simulink model "simlwrkuka_dynamic_dirdyn"  (R2014a)
settings: Solver=ode1  StartTime=0.0  StopTime=10.0  FixedStep=0.002  RelTol=1e-3
values from neighbouring files (symbols this model uses):
  dqi = [0;0;0;0;0;0;0]    [initial.m]
  qi = [pi/2;0;0;pi/2;0;pi/2;pi/6]    [initial.m]
settings Model: Creator=Admin  LastModifiedBy=faezeh

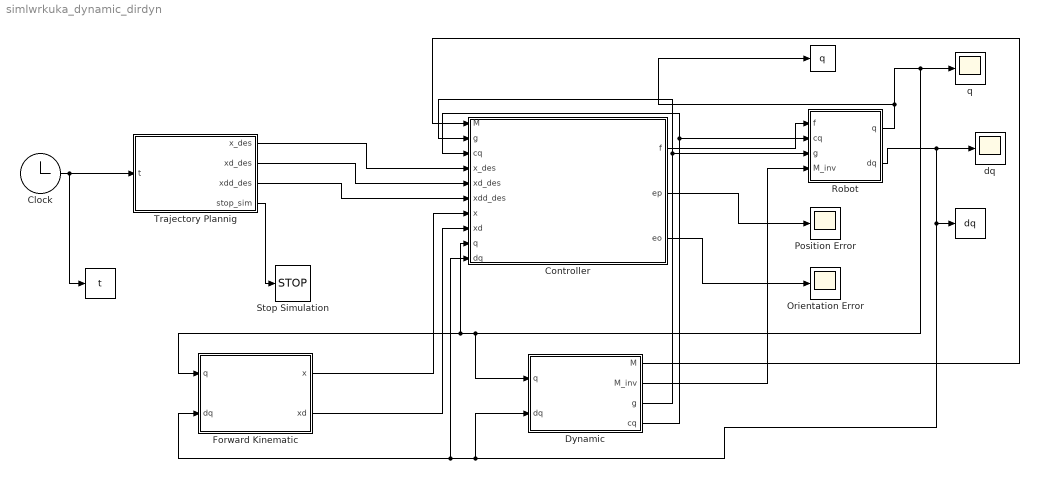
== system simlwrkuka_dynamic_dirdyn ==
  "  " : ToWorkspace  VariableName=q  SampleTime=-1
  "    " : ToWorkspace  VariableName=dq  SampleTime=-1
  "      " : ToWorkspace  VariableName=t  SampleTime=-1
  Clock : Clock
  Controller : MATLAB Function  TreatAsAtomicUnit=on
  Dynamic : MATLAB Function  TreatAsAtomicUnit=on
  Forward Kinematic : MATLAB Function  TreatAsAtomicUnit=on
  Orientation Error : Scope
      settings: SaveName=ScopeData2
  "Position Error " : Scope
  Robot : Subsystem
  Stop Simulation : Stop
  Trajectory Plannig : MATLAB Function  TreatAsAtomicUnit=on
  dq : Scope
      settings: SaveName=ScopeData3
  q : Scope
  wires:
  Clock/1 -> "      "/1, Trajectory Plannig/1(t)
  Trajectory Plannig/4(stop_sim) -> Stop Simulation/1
  Trajectory Plannig/3(xdd_des) -> Controller/6(xdd_des)
  Trajectory Plannig/2(xd_des) -> Controller/5(xd_des)
  Trajectory Plannig/1(x_des) -> Controller/4(x_des)
  Controller/1(f) -> Robot/1(f)
  Controller/2(ep) -> "Position Error "/1
  Controller/3(eo) -> Orientation Error/1
  Robot/1(q) -> Dynamic/1(q), Controller/9(q), Forward Kinematic/1(q), q/1, "  "/1
  Robot/2(dq) -> Dynamic/2(dq), Controller/10(dq), Forward Kinematic/2(dq), "    "/1, dq/1
  Forward Kinematic/1(x) -> Controller/7(x)
  Forward Kinematic/2(xd) -> Controller/8(xd)
  Dynamic/4(cq) -> Robot/2(cq), Controller/3(cq)
  Dynamic/3(g) -> Robot/3(g), Controller/2(g)
  Dynamic/1(M) -> Controller/1(M)
  Dynamic/2(M_inv) -> Robot/4(M_inv)

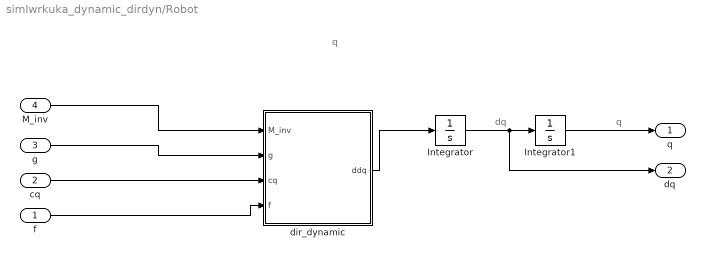
== system simlwrkuka_dynamic_dirdyn/Robot ==
  note: q
  note: q
  note: dq
  f : Inport
  cq : Inport  Port=2
  g : Inport  Port=3
  M_inv : Inport  Port=4
  Integrator : Integrator  InitialCondition=dqi
  Integrator1 : Integrator  InitialCondition=qi
  dir_dynamic : MATLAB Function  TreatAsAtomicUnit=on
  q : Outport
  dq : Outport  Port=2
  wires:
  f/1 -> dir_dynamic/4(f)
  dir_dynamic/1(ddq) -> Integrator/1
  Integrator/1 -> dq/1, Integrator1/1
  Integrator1/1 -> q/1
  g/1 -> dir_dynamic/2(g)
  M_inv/1 -> dir_dynamic/1(M_inv)
  cq/1 -> dir_dynamic/3(cq)

== matlab function simlwrkuka_dynamic_dirdyn/Controller ==
  data: M input; f output; g input; cq input; ep output; eo output; x_des input; xd_des input; xdd_des input; x input; xd input; q input; dq input
function [f,ep,eo] = command(M,g,cq,x_des,xd_des,xdd_des,x,xd,q,dq)
[J,Te]=jacobin(q(1),q(2),q(3),q(4),q(5),q(6),q(7));
Re=Te(1:3,1:3);
kp=15;
kd=10;
kpo=15;
eps=x(5:7);
eta=x(4);
eta_des=x_des(4);
eps_des=x_des(5:7);
S_eps=[0 -eps(3) eps(2); eps(3) 0 -eps(1);-eps(2) eps(1) 0];
eps_de=(eta*eps_des-eta_des*eps-S_eps*eps_des);
xd_com_o=xd_des(4:6)+kpo*Re*eps_de;
xd_com_p=xd_des(1:3)+kp*(x_des(1:3)-x(1:3));
Xd_com=[xd_com_p;xd_com_o];
f=M*pinv(J)*(xdd_des+kd*(xd_des-xd)+Xd_com-xd_des)+cq+g;
ep=x_des(1:3)-x(1:3);
eo=x_des(4:6)-x(4:6);

== matlab function simlwrkuka_dynamic_dirdyn/Trajectory Plannig ==
  data: t input; x_des output; xd_des output; xdd_des output; stop_sim output
function [x_des,xd_des,xdd_des,stop_sim] = fcn(t)
%linear trajectory
   xf=[0.085;-0.085;0.597];
   xi=[0;-0.39;0.61];
   L=norm(xf-xi);
   v_max=0.045; %v_max~L/7
   T=10;
   a_max=v_max^2/(T*v_max-L);
   stop_sim=0;
   sig=0;
   sigd=0;
   sigdd=0;

   Ts=v_max/a_max;
   if t<=Ts
   sig=a_max*t^2/2;
   sigd=a_max*t;
   sigdd=a_max;
   elseif t>Ts && t<=(T-Ts)
   sig=v_max*t-(v_max)^2/(2*a_max);
   sigd=v_max;
   sigdd=0;
   elseif t>(T-Ts) && t<=T
   sig=-a_max*(t-T)^2/2+v_max*T-(v_max)^2/a_max;
   sigd=-a_max*(t-T);
   sigdd=-a_max;
   else
       stop_sim=1;
   end
   R_des=[-0.866 -0.5 0;0.5 -0.866 0;0 0 1];
%    t_des=2.6180;f_des=0;s_des=0; 
%    euler_des=[t_des;f_des;s_des]; %Euler Representation
   eta_des=0.5*sqrt(R_des(1,1)+R_des(2,2)+R_des(3,3)+1);
   e_des=0.5*[sign(R_des(3,2)-R_des(2,3))*sqrt((R_des(1,1)-R_des(2,2)-R_des(3,3)+1));
              sign(R_des(1,3)-R_des(3,1))*sqrt((R_des(2,2)-R_des(3,3)-R_des(1,1)+1));
              sign(R_des(2,1)-R_des(1,2))*sqrt((R_des(3,3)-R_des(1,1)-R_des(2,2)+1))];
   Q_des=[eta_des;e_des]; %Unit Quaternion Representation
   x_des=[xi+sig*(xf-xi)/L;Q_des]; %7
   xd_des=[(xf-xi)/L*sigd;0;0;0]; %6
   xdd_des=[(xf-xi)/L*sigdd;0;0;0];

== matlab function simlwrkuka_dynamic_dirdyn/Robot/dir_dynamic ==
  data: M_inv input; g input; cq input; f input; ddq output
function ddq = dir_dyn(M_inv,g,cq,f)
 ddq=M_inv*(f-(cq+g));

== matlab function simlwrkuka_dynamic_dirdyn/Forward Kinematic ==
  data: q input; x output; xd output; dq input
function [x,xd]  = command(q,dq)
q1=q(1);q2=q(2);q3=q(3);q4=q(4);q5=q(5);q6=q(6);q7=q(7);
[J,Te]=jacobin(q1,q2,q3,q4,q5,q6,q7);
pe=Te(1:3,4);
Re=Te(1:3,1:3);
% f=atan2(R7(2,1),R7(1,1));
% t=atan2(-R7(3,1),sqrt(R7(3,2)^2+R7(3,3)^2));
% s=atan2(R7(3,2),R7(3,3)); 
% RPY=[s;t;f]; %RPY Representation
% f=atan2(Re(2,1),Re(1,1));
% t=atan2(-Re(3,1),sqrt(Re(3,2)^2+Re(3,3)^2));
% s=atan2(Re(3,2),Re(3,3));
% euler=[f;t;s];
% x=[p;euler];
eta=0.5*sqrt(Re(1,1)+Re(2,2)+Re(3,3)+1);
e=0.5*[sign(Re(3,2)-Re(2,3))*sqrt((Re(1,1)-Re(2,2)-Re(3,3)+1));
              sign(Re(1,3)-Re(3,1))*sqrt((Re(2,2)-Re(3,3)-Re(1,1)+1));
              sign(Re(2,1)-Re(1,2))*sqrt((Re(3,3)-Re(1,1)-Re(2,2)+1))];
Q=[eta;e]; %Unit Quaternion Representation
x=[pe;Q];
xd=J*dq;

== matlab function simlwrkuka_dynamic_dirdyn/Dynamic ==
  data: q input; M output; M_inv output; g output; cq output; dq input
function [M,M_inv,g,cq] = command(q,dq)
[M,M_inv,g]=kukalwrdynamic(q,dq);
C=0;
cq=C*dq;
